simulink library "RoomWifi"  (R2016b)
settings: Solver=VariableStepAuto  StartTime=0.0  StopTime=10.0  RelTol=1e-3
settings Model: Creator=sharo  LastModifiedBy=sharo

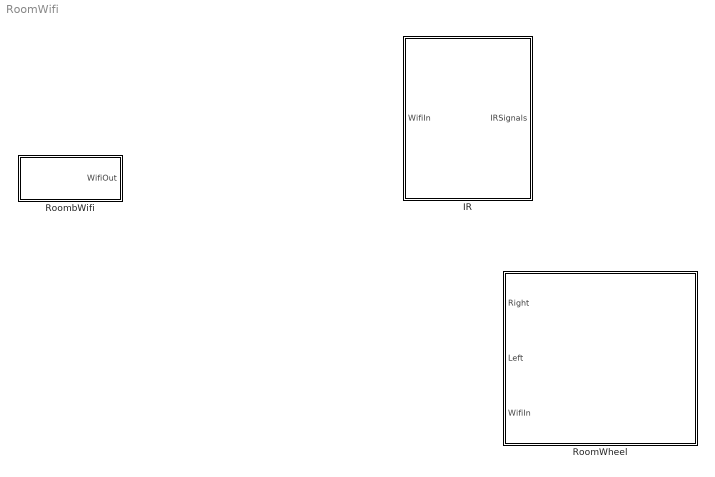
== system RoomWifi ==
  IR : Subsystem
  RoomWheel : Subsystem
  RoombWifi : Subsystem

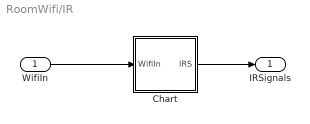
== system RoomWifi/IR ==
  WifiIn : Inport
  Chart : Stateflow chart  TreatAsAtomicUnit=on
  IRSignals : Outport
  wires:
  WifiIn/1 -> Chart/1(WifiIn)
  Chart/1(IRS) -> IRSignals/1

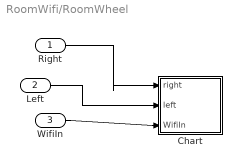
== system RoomWifi/RoomWheel ==
  Right : Inport
  Left : Inport  Port=2
  WifiIn : Inport  Port=3
  Chart : Stateflow chart  TreatAsAtomicUnit=on
  wires:
  Right/1 -> Chart/1(right)
  Left/1 -> Chart/2(left)
  WifiIn/1 -> Chart/3(WifiIn)

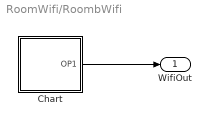
== system RoomWifi/RoombWifi ==
  Chart : Stateflow chart  TreatAsAtomicUnit=on
  "WifiOut " : Outport
  wires:
  Chart/1(OP1) -> "WifiOut "/1

== stateflow chart RoomWifi/IR/Chart ==
  state B
    entry,during:
    IRS = IRSense;
  (default) -> B
  data: x function_output; IRS output; WifiIn input
  function x = IRSense:
    | function x = IRSense
    | x = [0,0,0,0,0,0];
    | persistent obi
    | 
    | coder.extrinsic('evalin');
    | coder.extrinsic('RangeStateRoomba');
    | 
    | 
    | 
    | if isempty(obi);
    |     obi=evalin('base','so');
    | end
    | 
    | x = RangeStateRoomba(obi)

== stateflow chart RoomWifi/RoomWheel/Chart ==
  state C
    entry,during:
    WheelVelRoom(right,left);
  (default) -> C
  data: t function_input; u function_input; right input; left input; WifiIn input
  function WheelVelRoom(t,u):
    | function WheelVelRoom(t,u)
    | persistent obi;
    | coder.extrinsic('evalin')
    | 
    | coder.extrinsic('SetWheelVelRoomba');
    | 
    | 
    | if isempty(obi);
    |     obi=evalin('base','so');
    | end
    | 
    | SetWheelVelRoomba(obi,t,u)

== stateflow chart RoomWifi/RoombWifi/Chart ==
  state A
    entry, during:
    RWif
    OP1=0;
  (default) -> A
  data: OP1 output
  function RWif:
    | function RWif
    |  persistent obi;
    |  
    |  coder.extrinsic('assignin');
    |  coder.extrinsic('RoombaWifiInit');
    | 
    |  if isempty(obi)
    |        obi = RoombaWifiInit('10.0.0.1','full');
    |  end
    |  
    |  assignin('base','so',obi);
